simulink model "vrlights"  (Simulink 6.0)
settings: Solver=ode45  StartTime=0.0  StopTime=Inf  RelTol=1e-3
libraries: vrlib x1
settings Model: CovMetricSettings=d  Creator=Straka  LastModifiedBy=Houska  ExtModeTrigMode=oneshot  ExtModeArmWhenConnect=off
settings DataIOCC: LimitDataPoints=off  SaveOutput=off  SaveTime=off  SignalLoggingName=logsOut
settings OptimizationCC: BlockReduction=off  BooleanDataType=off
settings DebuggingCC: CheckExecutionContextPreStartOutputMsg=on  CheckExecutionContextRuntimeOutputMsg=on  SolverPrmCheckMsg=none
settings HardwareCC: TargetUnknown=on
settings ModelReferenceCC: UpdateModelReferenceTargets=IfOutOfDate
settings GRTTargetCC: LifeSpan=inf
settings SFSimCC: SFSimApplyToAllLibs=on  SFSimBuildMode=Incremental

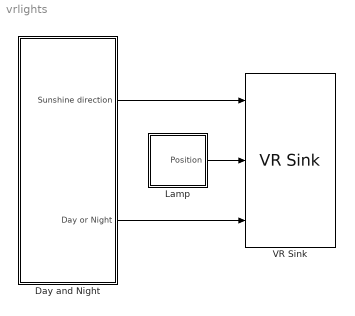
== system vrlights ==
  Day and Night : Subsystem  EnableExecutionContextPropagation=on
  Lamp : Subsystem  EnableExecutionContextPropagation=on
  VR Sink : vrlib/VR Sink  SampleTime=0.1  ViewEnable=on  RemoteChange=off  RemoteView=off  FieldsWritten=Sun.direction.3.1.double#Lamp.location.3.1.double#Lamp.on.1.1.logical  WorldFileName=vrlights.wrl  AutoView=on
  wires:
  Lamp/1(Position) -> VR Sink/2
  Day and Night/2(Day or Night) -> VR Sink/3
  Day and Night/1(Sunshine direction) -> VR Sink/1

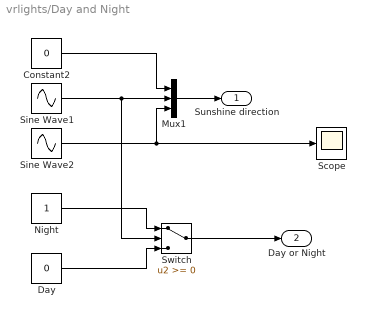
== system vrlights/Day and Night ==
  Constant2 : Constant  Value=0
  Day : Constant  Value=0
  Mux1 : Mux  Inputs=3
  Night : Constant
  Scope : Scope
  Sine Wave1 : Sin  Frequency=0.03  Phase=-1.57  SampleTime=0
  Sine Wave2 : Sin  Frequency=0.03  SampleTime=0
  Switch : Switch  InputSameDT=on
  Sunshine direction : Outport
  Day or Night : Outport  Port=2
  wires:
  Constant2/1 -> Mux1/1
  Mux1/1 -> Sunshine direction/1
  Night/1 -> Switch/1
  Day/1 -> Switch/3
  Sine Wave1/1 -> Mux1/2, Switch/2
  Sine Wave2/1 -> Mux1/3, Scope/1
  Switch/1 -> Day or Night/1

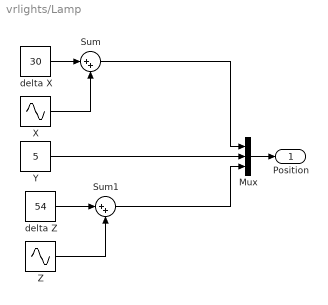
== system vrlights/Lamp ==
  Mux : Mux  Inputs=3
  Sum : Sum  Inputs=|++  SaturateOnIntegerOverflow=on  InputSameDT=on
  Sum1 : Sum  Inputs=|++  SaturateOnIntegerOverflow=on  InputSameDT=on
  X : Sin  Amplitude=20  Frequency=0.065  SampleTime=0
  Y : Constant  Value=5
  Z : Sin  Amplitude=24  Frequency=0.05  SampleTime=0
  delta X : Constant  Value=30
  delta Z : Constant  Value=54
  Position : Outport
  wires:
  delta X/1 -> Sum/1
  Y/1 -> Mux/2
  delta Z/1 -> Sum1/1
  Mux/1 -> Position/1
  Sum1/1 -> Mux/3
  Sum/1 -> Mux/1
  Z/1 -> Sum1/2
  X/1 -> Sum/2
